simulink library "arsenal"  (R2024b)
settings: Solver=VariableStepAuto  StartTime=0.0  StopTime=10.0  RelTol=1e-3
libraries: fl_lib x15, simulink x2, sdl_lib x2
settings Model: Creator=upattacini  LastModifiedBy=upattacini

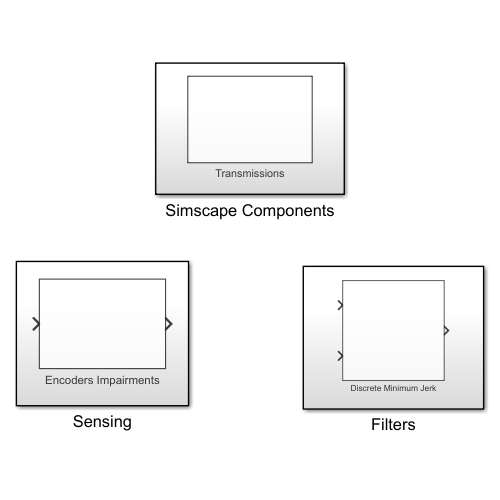
[thumbnail: Simulink's stored preview of the top-level diagram]
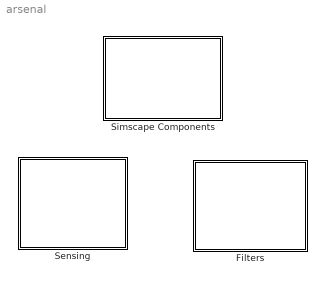
== system arsenal ==
  Filters : Subsystem
  Sensing : Subsystem
  Simscape Components : Subsystem

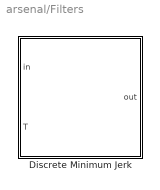
== system arsenal/Filters ==
  Discrete Minimum Jerk : Subsystem  mask(Minimum Jerk Filter){Ts=0.001}
      mask prompts: Ts "Sample time (s)"
      mask help:
      | Apply quasi-minimum jerk filtering to the input.
      | The filter reactivity can be adjusted via the input T, which specifies the rise-time.

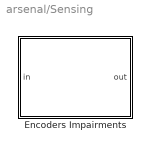
== system arsenal/Sensing ==
  Encoders Impairments : Subsystem  mask(Encoders Impairments){bit_resolution=14, bit_noise=2, seed=0, Ts=0.001}
      mask prompts: bit_resolution "Bits or resolution"; bit_noise "Bits of noise"; Ts "Sample time (s)"
      mask help:
      | Simulate the impairments underlying the encoders readouts.
      | In particular, the block simulates the effects of quantization and noise.

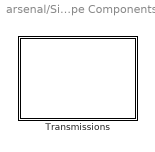
== system arsenal/Simscape Components ==
  Transmissions : Subsystem

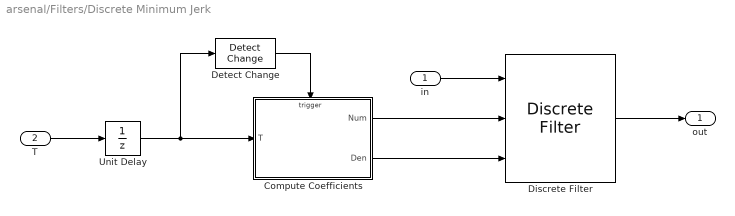
== system arsenal/Filters/Discrete Minimum Jerk ==
  in : Inport  PortDimensions=1
  T : Inport  Port=2  PortDimensions=1
  Compute Coefficients : Subsystem
  Detect Change : simulink/Logic and Bit Operations/Detect Change  vinit=0  OutDataTypeStr=uint8
  Discrete Filter : DiscreteFilter  NumeratorSource=Input port  DenominatorSource=Input port  a0EqualsOne=on
      settings: InputPortMap=u0,p1,p3
  Unit Delay : UnitDelay  SampleTime=Ts  HasFrameUpgradeWarning=on
  out : Outport  PortDimensions=1
  wires:
  in/1 -> Discrete Filter/1
  Discrete Filter/1 -> out/1
  Unit Delay/1 -> Compute Coefficients/1(T), Detect Change/1
  Detect Change/1 -> Compute Coefficients/Trigger
  Compute Coefficients/1(Num) -> Discrete Filter/2
  T/1 -> Unit Delay/1
  Compute Coefficients/2(Den) -> Discrete Filter/3

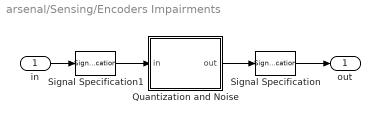
== system arsenal/Sensing/Encoders Impairments ==
  in : Inport
  Quantization and Noise : Subsystem  mask{bit_resolution=bit_resolution, bit_noise=bit_noise, seed=0, Ts=Ts}
      mask prompts: bit_resolution "Resolution bits"; bit_noise "Noise bits"; Ts "Sample time (s)"
      settings: PortSchema="{\"entries\":[{\"content\":{\"sides\":[{\"content\":{\"connectorIds\":[\"Out1\"]},\"type\":\"ConnectorPlacement.EquallySpacedRectSide\",\"uuid\":\"5c60203e-1477-4c63-bf85-2a9264896243\"},{\"content\":{\"connectorIds\":[\"In1\"],\"side\":\"RIGHT\"},\"type\":\"ConnectorPlacement.EquallySpacedRectSide\",\"uuid\":\"fde9215e-0eee-4b90-b3d3-bc5e0578faf0\"},{\"content\":{\"side\":\"TOP\"},\"type\":\"ConnectorPlacement.EquallySpacedRectSide\",\"uuid\":\"75472767-9856-4b99-a0f4-bd856ef58e73\"}]},\"type\":\"ConnectorPlacement.EquallySpacedConnector\",\"uuid\":\"089ac2bf-9317-43ab-ab34-2d9e1bbbe948\"}],\"packageUris\":[\"http://schema.mathworks.com/mf0/Connector/R2020b\"],\"version\":\"1.0\"}"
  Signal Specification : SignalSpecification  Unit=deg
  Signal Specification1 : SignalSpecification  Unit=deg
  out : Outport
  wires:
  in/1 -> Signal Specification1/1
  Quantization and Noise/1(out) -> Signal Specification/1
  Signal Specification/1 -> out/1
  Signal Specification1/1 -> Quantization and Noise/1(in)

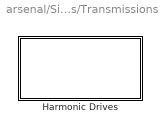
== system arsenal/Simscape Components/Transmissions ==
  Harmonic Drives : Subsystem

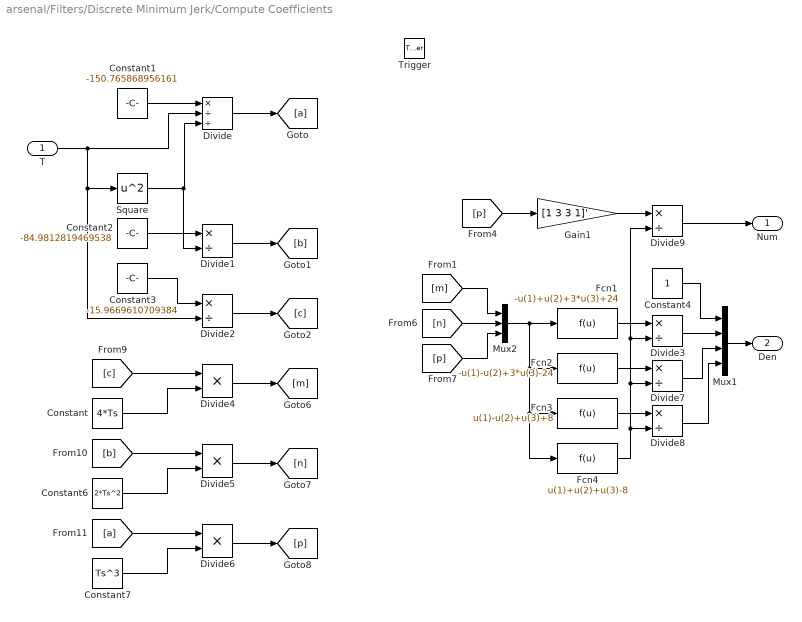
== system arsenal/Filters/Discrete Minimum Jerk/Compute Coefficients ==
  T : Inport
  Trigger : TriggerPort  VariantControl=(inherit)  PortDimensions=1
  Constant : Constant  Value=4*Ts
  Constant1 : Constant  Value=-150.765868956161
  Constant2 : Constant  Value=-84.9812819469538
  Constant3 : Constant  Value=-15.9669610709384
  Constant4 : Constant
  Constant6 : Constant  Value=2*Ts^2
  Constant7 : Constant  Value=Ts^3
  Divide : Product  Inputs=*//
  Divide{1..3,7..9} (6 alike) : Product  Inputs=*/
  Divide4 : Product  Inputs=**
  Divide5 : Product  Inputs=**
  Divide6 : Product  Inputs=**
  Fcn1 : Fcn  Expr=-u(1)+u(2)+3*u(3)+24
  Fcn2 : Fcn  Expr=-u(1)-u(2)+3*u(3)-24
  Fcn3 : Fcn  Expr=u(1)-u(2)+u(3)+8
  Fcn4 : Fcn  Expr=u(1)+u(2)+u(3)-8
  Gain1 : Gain  Gain=[1 3 3 1]'
  Mux1 : Mux
  Mux2 : Mux  Inputs=3
  Square : Math  Operator=square
  Num : Outport  InitialOutput=[0 0 0 0]
  Den : Outport  Port=2  InitialOutput=[1 0 0 0]'
  wires:
  Divide9/1 -> Num/1
  Gain1/1 -> Divide9/1
  Fcn4/1 -> Divide3/2, Divide9/2, Divide7/2, Divide8/2
  Fcn3/1 -> Divide8/1
  Fcn2/1 -> Divide7/1
  Divide8/1 -> Mux1/4
  Divide7/1 -> Mux1/3
  Divide3/1 -> Mux1/2
  Fcn1/1 -> Divide3/1
  Mux2/1 -> Fcn1/1, Fcn2/1, Fcn3/1, Fcn4/1
  [p] -> Mux2/3
  [n] -> Mux2/2
  [m] -> Mux2/1
  Constant7/1 -> Divide6/2
  [a] -> Divide6/1
  Divide6/1 -> [p]
  Divide5/1 -> [n]
  [b] -> Divide5/1
  Constant6/1 -> Divide5/2
  Constant/1 -> Divide4/2
  [c] -> Divide4/1
  Divide4/1 -> [m]
  Mux1/1 -> Den/1
  Constant4/1 -> Mux1/1
  Divide/1 -> [a]
  Square/1 -> Divide/3, Divide1/2
  Constant3/1 -> Divide2/1
  Constant2/1 -> Divide1/1
  [p] -> Gain1/1
  Divide2/1 -> [c]
  T/1 -> Divide/2, Square/1, Divide2/2
  Divide1/1 -> [b]
  Constant1/1 -> Divide/1

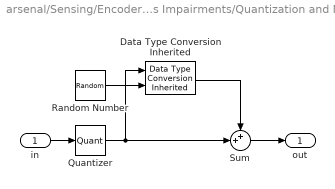
== system arsenal/Sensing/Encoders Impairments/Quantization and Noise ==
  in : Inport
  Data Type Conversion Inherited : simulink/Signal Attributes/Data Type Conversion Inherited  ConvertRealWorld=Real World Value  DoSatur=off
  Quantizer : Quantizer  QuantizationInterval=360/2^bit_resolution
  Random Number : RandomNumber  Variance=((360/2^bit_resolution)*(2^bit_noise-1) * (1/3))^2  Seed=seed  SampleTime=Ts
  Sum : Sum  Inputs=++|
  out : Outport
  wires:
  Quantizer/1 -> Data Type Conversion Inherited/1, Sum/2
  Random Number/1 -> Data Type Conversion Inherited/2
  in/1 -> Quantizer/1
  Sum/1 -> out/1
  Data Type Conversion Inherited/1 -> Sum/1

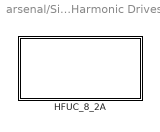
== system arsenal/Simscape Components/Transmissions/Harmonic Drives ==
  HFUC_8_2A : Subsystem

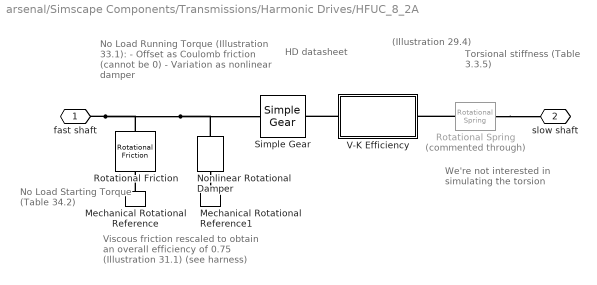
== system arsenal/Simscape Components/Transmissions/Harmonic Drives/HFUC_8_2A ==
  note: No Load Starting Torque
      | (Table 34.2)
  note: No Load Running Torque (Illustration 33.1):
      | - Offset as Coulomb friction (cannot be 0)
      | - Variation as nonlinear damper
  note: Torsional stiffness
      | (Table 3.3.5)
  note: Viscous friction rescaled to obtain an
      | overall efficiency of 0.75 (Illustration 31.1)
      | (see harness)
  note: (Illustration 29.4)
  note: HD datasheet
  note: We're not interested in
      | simulating the torsion
  Mechanical Rotational Reference : fl_lib/Mechanical/Rotational Elements/Mechanical Rotational Reference
  Mechanical Rotational Reference1 : fl_lib/Mechanical/Rotational Elements/Mechanical Rotational Reference
  Nonlinear Rotational Damper : sdl_lib/Couplings & Drives/Springs & Dampers/Nonlinear Rotational Damper  parameterization=sdl.enum.polynomialTLU.tlu  symmetry=sdl.enum.symmetry.symmetric  coefficient_vector=[.0001, 0, 1e-05, 0, 1e-06] N*m*s/rad  positive_coefficient_vector=[.0001, 0, 1e-05, 0, 1e-06] N*m*s/rad  negative_coefficient_vector=[.001, -1e-05, .0001, 0, 0] N*m*s/rad  angular_velocity_vector=[-3500, -2000, -1000, -500, 500, 1000, 2000, 3500] rpm  torque_vector=[-0.7, -0.2, -0.1, 0, 0, 0.1, 0.2, 0.7]*0.5 N*cm  interp_method=simscape.enum.interpolation.linear  extrap_method=simscape.enum.extrapolation.nearest
      settings: InternalSimscapePortConfiguration="{\"Bottom\":[],\"Left\":[{\"id\":\"R\",\"label\":\"R\",\"type\":\"foundation.mechanical.rotational.rotational\"}],\"Right\":[{\"id\":\"C\",\"label\":\"C\",\"type\":\"foundation.mechanical.rotational.rotational\"}],\"Top\":[]}"
  Rotational Friction : fl_lib/Mechanical/Rotational Elements/Rotational Friction  brkwy_trq=0.59 N*cm  brkwy_vel=0.001 rad/s  Col_trq=0.3*0.5 N*cm  visc_coef=0 N*cm/rpm  w_specify=off  w_priority=None  w=0 rad/s  w_nominal_specify=off  w_nominal_value=1  w_nominal_unit=rad/s  t_specify=off  t_priority=None  t=0 N*m  t_nominal_specify=off  t_nominal_value=1  t_nominal_unit=N*m
  Rotational Spring : fl_lib/Mechanical/Rotational Elements/Rotational Spring  Commented=through  spr_rate=1000 N*m/rad  w_specify=off  w_priority=None  w=0 rad/s  w_nominal_specify=off  w_nominal_value=1  w_nominal_unit=rad/s  t_specify=off  t_priority=None  t=0 N*m  t_nominal_specify=off  t_nominal_value=1  t_nominal_unit=N*m  phi_specify=off  phi_priority=High  phi=0 rad  phi_nominal_specify=off  phi_nominal_value=1  phi_nominal_unit=rad
  Simple Gear : sdl_lib/Gears/Simple Gear  ratio=100  rotation_direction=sdl.enum.shaftOutputDirection.opposite  friction_model=sdl.enum.gear_efficiencies_load.off  T_noload=0.1 N*m  T_nom=5 N*m  efficiency_nom=0.8  efficiency=1  temperature_TLU=[280, 300, 320] K  load_TLU=[1, 5, 10] N*m  efficiency_TLU=[.95, .9, .85]  efficiency_TLU2=[.85, .8, .75; .95, .9, .85; .85, .8, .7]  w_thr=0.01 rad/s  pwr_thr=0.001 W  enable_backlash=false  hardstop_model=simscape.enum.hardstop.smooth  backlash_distance=1e-3 mm  r_base=0.1 m  transition=1e-4 mm  backlash_stiffness=1e6 N/m  backlash_damping=1e3 N*s/m  coeff_rest=0.7  v_tol=0.001 m/s  f_tol=0.001 N  mu_visc=[0, 0] N*cm*s/rad  thermal_mass=50 J/K  temperature_specify=off  temperature_priority=High  temperature=300 K  temperature_nominal_specify=off  temperature_nominal_value=1  temperature_nominal_unit=K  x_backlash_specify=off  x_backlash_priority=None  x_backlash=0 mm  x_backlash_nominal_specify=off  x_backlash_nominal_value=1  x_backlash_nominal_unit=mm  f_hardstop_specify=off  f_hardstop_priority=None  f_hardstop=0 N  f_hardstop_nominal_specify=off  f_hardstop_nominal_value=1  f_hardstop_nominal_unit=N  v_backlash_specify=off  v_backlash_priority=None  v_backlash=0 m/s  v_backlash_nominal_specify=off  v_backlash_nominal_value=1  v_backlash_nominal_unit=m/s
  V-K Efficiency : Subsystem
  fast shaft : PMIOPort  Side=Left  ConnectionType=Connection: foundation.mechanical.rotational.rotational
  slow shaft : PMIOPort  Port=2  Side=Right  ConnectionType=Connection: foundation.mechanical.rotational.rotational
  connections:
  V-K Efficiency/LConn1 -- Simple Gear/RConn1
  Rotational Spring/LConn1 -- V-K Efficiency/RConn1
  Rotational Spring/RConn1 -- slow shaft/RConn1
  Nonlinear Rotational Damper/RConn1 -- Mechanical Rotational Reference1/LConn1
  Mechanical Rotational Reference/LConn1 -- Rotational Friction/RConn1
  fast shaft/RConn1 -- Rotational Friction/LConn1 -- Nonlinear Rotational Damper/LConn1 -- Simple Gear/LConn1

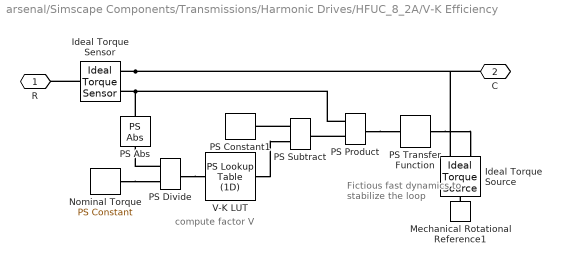
== system arsenal/Simscape Components/Transmissions/Harmonic Drives/HFUC_8_2A/V-K Efficiency ==
  note: Fictious fast dynamics
      | to stabilize the loop
  note: compute
      | factor V
  Ideal Torque Sensor : fl_lib/Mechanical/Mechanical Sensors/Ideal Torque Sensor
  Ideal Torque Source : fl_lib/Mechanical/Mechanical Sources/Ideal Torque Source
  Mechanical Rotational Reference1 : fl_lib/Mechanical/Rotational Elements/Mechanical Rotational Reference
  Nominal Torque : fl_lib/Physical Signals/Sources/PS Constant  constant=2.4 N*m
  PS Abs : fl_lib/Physical Signals/Nonlinear Operators/PS Abs
      settings: InternalSimscapePortConfiguration="{\"Bottom\":[],\"Left\":[{\"id\":\"I\",\"label\":\"\",\"type\":\"input\"}],\"Right\":[{\"id\":\"O\",\"label\":\"\",\"type\":\"output\"}],\"Top\":[]}"
  PS Constant1 : fl_lib/Physical Signals/Sources/PS Constant  constant=1
  PS Divide : fl_lib/Physical Signals/Functions/PS Divide
  PS Product : fl_lib/Physical Signals/Functions/PS Product
  PS Subtract : fl_lib/Physical Signals/Functions/PS Subtract
  PS Transfer Function : fl_lib/Physical Signals/Linear Operators/PS Transfer Function  transfer_function_type=foundation.enum.transfer_function_type.lag  T=1e-6 s  T1=2 s  T2=1 s  reset_method=foundation.enum.IntegratorResetSpec.None  initial_condition_spec=foundation.enum.IntegratorICSpec.Internal  y0=0 N*m
      settings: InternalSimscapePortConfiguration="{\"Bottom\":[],\"Left\":[{\"id\":\"U\",\"label\":\"\",\"type\":\"input\"}],\"Right\":[{\"id\":\"Y\",\"label\":\"\",\"type\":\"output\"}],\"Top\":[]}"
  V-K LUT : fl_lib/Physical Signals/Lookup Tables/PS Lookup Table (1D)  x=[0.1, 0.2, 0.4, 0.6, 0.8, 1]  f=[0.45, 0.65, 0.85, 0.95, 0.99, 1]  interp_method=simscape.enum.interpolation.linear  extrap_method=simscape.enum.extrapolation.nearest
  R : PMIOPort  Side=Left
  C : PMIOPort  Port=2  Side=Right
  connections:
  PS Transfer Function/RConn1 -- Ideal Torque Source/RConn1
  Mechanical Rotational Reference1/LConn1 -- Ideal Torque Source/LConn1
  PS Product/RConn1 -- PS Transfer Function/LConn1
  PS Product/LConn2 -- PS Subtract/RConn1
  V-K LUT/RConn1 -- PS Subtract/LConn2
  PS Subtract/LConn1 -- PS Constant1/RConn1
  PS Divide/RConn1 -- V-K LUT/LConn1
  Nominal Torque/RConn1 -- PS Divide/LConn2
  Ideal Torque Sensor/RConn1 -- Ideal Torque Source/RConn2 -- C/RConn1
  Ideal Torque Sensor/LConn1 -- R/RConn1
  Ideal Torque Sensor/RConn2 -- PS Product/LConn1 -- PS Abs/LConn1
  PS Divide/LConn1 -- PS Abs/RConn1
